simulink library "rotation_resistance"  (R2020b)
settings: Solver=VariableStepAuto  StartTime=0.0  StopTime=10.0  RelTol=1e-3
values from neighbouring files (symbols this model uses):
  Jg = 0.14    [Projektskript.m]    (also in init.m)
  rrad = 0.3    [Projektskript.m]    (also in init.m)
settings Model: Creator=janbantle  LastModifiedBy=Johnathy

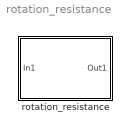
== system rotation_resistance ==
  rotation_resistance : Subsystem

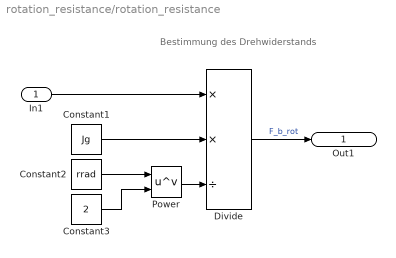
== system rotation_resistance/rotation_resistance ==
  note: Bestimmung des Drehwiderstands
  In1 : Inport
  Constant1 : Constant  Value=Jg
  Constant2 : Constant  Value=rrad
  Constant3 : Constant  Value=2
  Divide : Product  Inputs=**/
  Power : Math  Operator=pow  SaturateOnIntegerOverflow=on
  Out1 : Outport
  wires:
  Constant3/1 -> Power/2
  Constant1/1 -> Divide/2
  Power/1 -> Divide/3
  Constant2/1 -> Power/1
  Divide/1 -> Out1/1  "F_b_rot"
  In1/1 -> Divide/1
